simulink model "model"  (R2022a)
settings: Solver=ode4  StartTime=0.0  StopTime=45  FixedStep=5e-3  RelTol=1e-3
values from neighbouring files (symbols this model uses):
  emin = 0.1    [simulate.m]
  poseG = [0,0,0]    [simulate.m]
  poseR0 = poseR0_list(i,:)    [simulate.m]
settings Model: Creator=mateu  LastModifiedBy=mateu

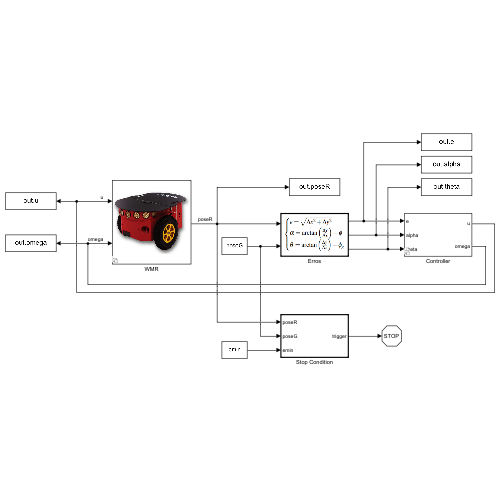
[thumbnail: Simulink's stored preview of the top-level diagram]
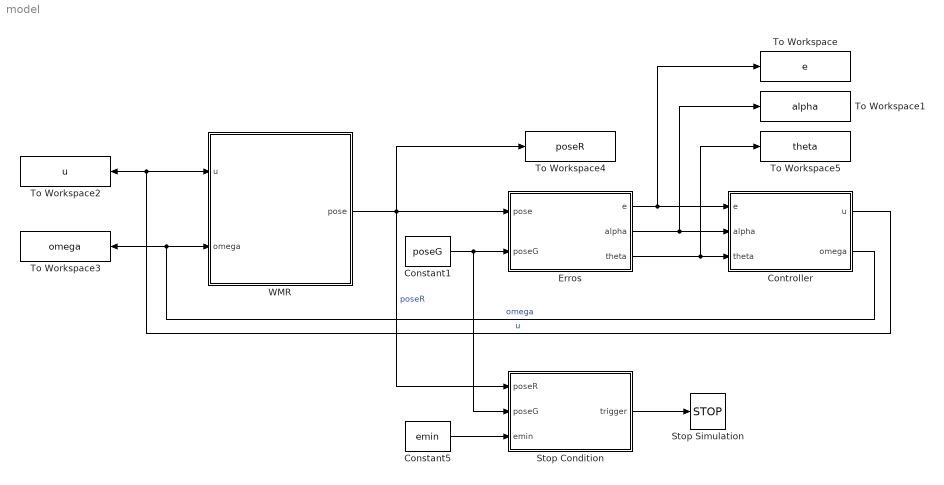
== system model ==
  Constant1 : Constant  Value=poseG
  Constant5 : Constant  Value=emin
  Controller : Subsystem  Variant=on
      mask Display: image('$imagefile'); % Use "Edit Image" on toolstrip to change.
  Erros : MATLAB Function  TreatAsAtomicUnit=on
  Stop Condition : MATLAB Function  TreatAsAtomicUnit=on
  Stop Simulation : Stop
  To Workspace : ToWorkspace  VariableName=e  SaveFormat=Timeseries  SampleTime=-1
  To Workspace1 : ToWorkspace  VariableName=alpha  SaveFormat=Timeseries  SampleTime=-1
  To Workspace2 : ToWorkspace  VariableName=u  SaveFormat=Timeseries  SampleTime=-1
  To Workspace3 : ToWorkspace  VariableName=omega  SaveFormat=Timeseries  SampleTime=-1
  To Workspace4 : ToWorkspace  VariableName=poseR  SaveFormat=Timeseries  SampleTime=-1
  To Workspace5 : ToWorkspace  VariableName=theta  SaveFormat=Timeseries  SampleTime=-1
  WMR : Subsystem  Variant=on
      mask Display: image('$imagefile'); % Use "Edit Image" on toolstrip to change.
  wires:
  WMR/1(pose) -> To Workspace4/1, Stop Condition/1(poseR), Erros/1(pose)  "poseR"
  Erros/1(e) -> To Workspace/1, Controller/1(e)
  Erros/2(alpha) -> To Workspace1/1, Controller/2(alpha)
  Erros/3(theta) -> To Workspace5/1, Controller/3(theta)
  Stop Condition/1(trigger) -> Stop Simulation/1
  Constant5/1 -> Stop Condition/3(emin)
  Constant1/1 -> Stop Condition/2(poseG), Erros/2(poseG)
  Controller/2(omega) -> WMR/2(omega), To Workspace3/1  "omega"
  Controller/1(u) -> WMR/1(u), To Workspace2/1  "u"

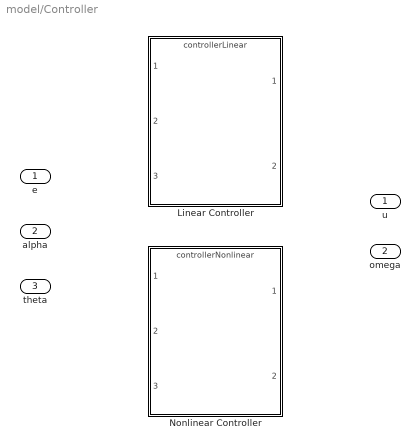
== system model/Controller ==
  e : Inport
  alpha : Inport  Port=2
  theta : Inport  Port=3
  Linear Controller : ModelReference  DisableCoverage=on  ModelNameDialog=controllerLinear  VariantControl=CONTROL_LINEAR  ModelReferenceVersion=1.1
  Nonlinear Controller : ModelReference  ModelNameDialog=controllerNonlinear  VariantControl=CONTROL_NONLINEAR  ModelReferenceVersion=1.1
  u : Outport
  omega : Outport  Port=2

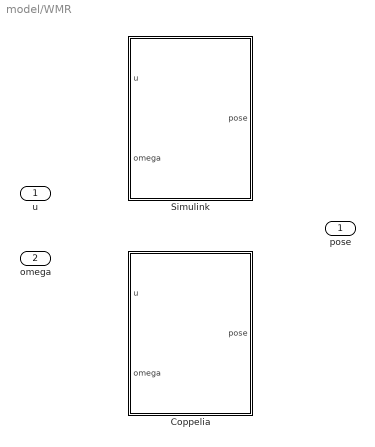
== system model/WMR ==
  u : Inport
  omega : Inport  Port=2
  Coppelia : Subsystem  VariantControl=UNICYCLE_COPPELIA
  Simulink : Subsystem  VariantControl=UNICYCLE_SIMULINK
  pose : Outport

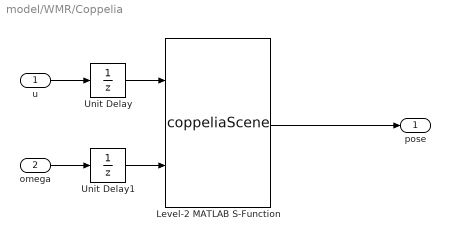
== system model/WMR/Coppelia ==
  u : Inport
  omega : Inport  Port=2
  Level-2 MATLAB S-Function : M-S-Function  FunctionName=coppeliaScene  Parameters=poseR0
  Unit Delay : UnitDelay  SampleTime=-1  HasFrameUpgradeWarning=on
  Unit Delay1 : UnitDelay  SampleTime=-1  HasFrameUpgradeWarning=on
  pose : Outport
  wires:
  u/1 -> Unit Delay/1
  omega/1 -> Unit Delay1/1
  Level-2 MATLAB S-Function/1 -> pose/1
  Unit Delay/1 -> Level-2 MATLAB S-Function/1
  Unit Delay1/1 -> Level-2 MATLAB S-Function/2

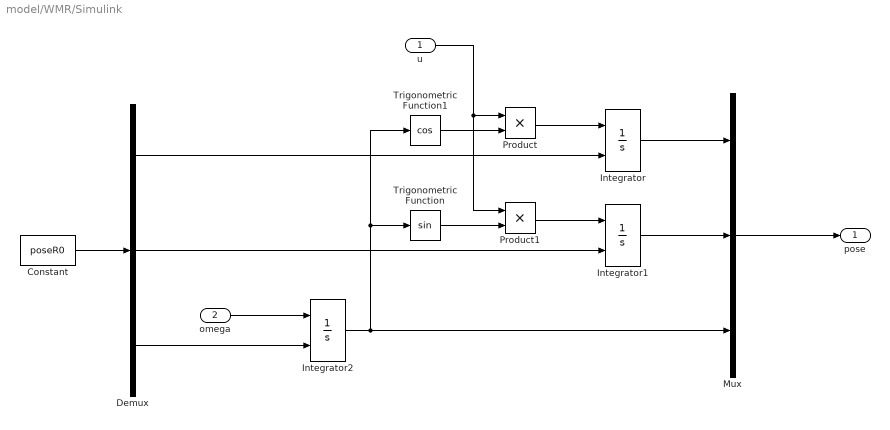
== system model/WMR/Simulink ==
  u : Inport
  omega : Inport  Port=2
  Constant : Constant  Value=poseR0
  Demux : Demux  Outputs=3
  Integrator : Integrator  InitialConditionSource=external
  Integrator1 : Integrator  InitialConditionSource=external
  Integrator2 : Integrator  InitialConditionSource=external
  Mux : Mux  Inputs=3
  Product : Product
  Product1 : Product
  Trigonometric Function : Trigonometry
  Trigonometric Function1 : Trigonometry  Operator=cos
  pose : Outport
  wires:
  Demux/3 -> Integrator2/2
  Constant/1 -> Demux/1
  Mux/1 -> pose/1
  Integrator2/1 -> Trigonometric Function1/1, Trigonometric Function/1, Mux/3
  Demux/1 -> Integrator/2
  omega/1 -> Integrator2/1
  Product1/1 -> Integrator1/1
  Product/1 -> Integrator/1
  Trigonometric Function1/1 -> Product/2
  Trigonometric Function/1 -> Product1/2
  Demux/2 -> Integrator1/2
  u/1 -> Product/1, Product1/1
  Integrator1/1 -> Mux/2
  Integrator/1 -> Mux/1

== matlab function model/Erros ==
  settings: updateMethod=DISCRETE  sampleTime=0.05
  data: pose input; e output; poseG input; alpha output; theta output
function [e,alpha,theta] = errors(pose,poseG)

deltaX = poseG(1)-pose(1); deltaY = poseG(2)-pose(2);
phi = pose(3); phiG = poseG(3);

e = sqrt(deltaX^2 + deltaY^2);
alpha = atan2(deltaY,deltaX) - phi;
theta = atan2(deltaY,deltaX) - phiG;

== matlab function model/Stop Condition ==
  data: poseR input; trigger output; poseG input; emin input
function trigger = stopCondition(poseR,poseG,emin)

trigger = sqrt(sum((poseG-poseR).^2)) <= emin;
